simulink model "Position_Control_Pre"  (R2015b)
settings: Solver=VariableStepAuto  StartTime=0.0  StopTime=1  RelTol=1e-3
settings Model: Creator=TOSHIBA  LastModifiedBy=TOSHIBA

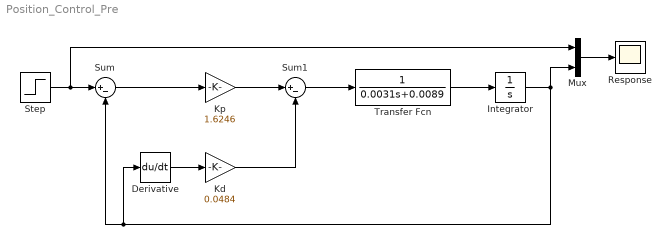
== system Position_Control_Pre ==
  Derivative : Derivative
  Integrator : Integrator
  Kd : Gain  Gain=0.0484
  Kp : Gain  Gain=1.6246
  Mux : Mux  Inputs=2
  Response : Scope
  Step : Step  Time=0  After=pi/18  SampleTime=0
  Sum : Sum  Inputs=|+-
  Sum1 : Sum  Inputs=|+-
  Transfer Fcn : TransferFcn  Denominator=[0.0031 0.0089]
  wires:
  Derivative/1 -> Kd/1
  Step/1 -> Mux/1, Sum/1
  Sum/1 -> Kp/1
  Kp/1 -> Sum1/1
  Sum1/1 -> Transfer Fcn/1
  Transfer Fcn/1 -> Integrator/1
  Integrator/1 -> Mux/2, Derivative/1, Sum/2
  Kd/1 -> Sum1/2
  Mux/1 -> Response/1
